simulink model "test_10gbe_mux_with_buffers"  (Simulink 6.2)
settings: Solver=ode45  StartTime=0.0  StopTime=4000  RelTol=1e-3
undefined symbols (not defined in the file): BEE2_usr
libraries: xbsIndex_r3 x551, xps_library x35, casper_library x16
(part 1 of 3)
settings Model: LastModifiedBy=dsp
settings DebuggingCC: SolverPrmCheckMsg=warning

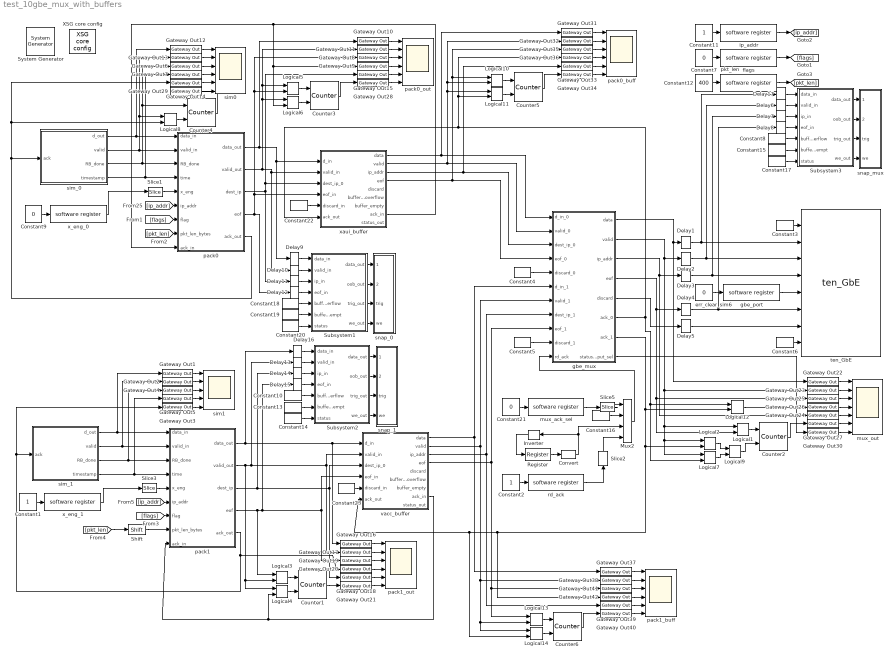
== system test_10gbe_mux_with_buffers ==
  " System Generator" : xbsIndex_r3/ System Generator  Tag=genX  xilinxfamily=Virtex2P  part=xc2vp70  speed=-7  package=ff1704  synthesis_tool=XST  directory=./test_mp_ub1/sysgen  testbench=off  simulink_period=1  sysclk_period=4.878  incr_netlist=off  trim_vbits=Everywhere in SubSystem  dbl_ovrd=According to Block Masks  core_generation=According to Block Masks  run_coregen=off  deprecated_control=off  eval_field=0
      settings: AttributesFormatString=System\nGenerator
  Constant1 : Constant
  Constant{3..5,8,10,13,15,18..19,22..23} (11 alike) : xbsIndex_r3/Constant  const=0  equ=P=C  arith_type=Boolean  n_bits=32  bin_pt=0  opselect=C  inp2=PCIN>>17  opr=+  inp1=P  carry=CIN  iostate=0  explicit_period=on  period=1  dbl_ovrd=off
  Constant11 : Constant
  Constant12 : Constant  Value=400
  Constant14 : xbsIndex_r3/Constant  const=0  equ=P=C  arith_type=Unsigned  n_bits=9  bin_pt=0  opselect=C  inp2=PCIN>>17  opr=+  inp1=P  carry=CIN  iostate=0  explicit_period=on  period=1  dbl_ovrd=off
  Constant16 : xbsIndex_r3/Constant  const=1  equ=P=C  arith_type=Boolean  n_bits=1  bin_pt=0  opselect=C  inp2=PCIN>>17  opr=+  inp1=P  carry=CIN  iostate=0  explicit_period=on  period=1  dbl_ovrd=off
  Constant17 : xbsIndex_r3/Constant  const=0  equ=P=C  arith_type=Unsigned  n_bits=9  bin_pt=0  opselect=C  inp2=PCIN>>17  opr=+  inp1=P  carry=CIN  iostate=0  explicit_period=on  period=1  dbl_ovrd=off
  Constant2 : Constant
  Constant20 : xbsIndex_r3/Constant  const=0  equ=P=C  arith_type=Unsigned  n_bits=9  bin_pt=0  opselect=C  inp2=PCIN>>17  opr=+  inp1=P  carry=CIN  iostate=0  explicit_period=on  period=1  dbl_ovrd=off
  Constant21 : Constant  Value=0
  Constant6 : xbsIndex_r3/Constant  const=1  equ=P=C  arith_type=Boolean  n_bits=32  bin_pt=0  opselect=C  inp2=PCIN>>17  opr=+  inp1=P  carry=CIN  iostate=0  explicit_period=on  period=1  dbl_ovrd=off
  Constant7 : Constant  Value=0
  Constant9 : Constant  Value=0
  Convert : xbsIndex_r3/Convert  arith_type=Boolean  n_bits=1  bin_pt=6  quantization=Truncate  overflow=Wrap  latency=0  explicit_period=off  period=1  dbl_ovrd=off  show_param=off  inserted_by_tool=off  pipeline=off
      settings: xl_area=[0, 0, 0, 0, 0, 0, 0]
  Counter{1..6} (6 alike) : xbsIndex_r3/Counter  cnt_type=Free Running  n_bits=8  bin_pt=0  arith_type=Unsigned  start_count=0  cnt_to=Inf  cnt_by_val=1  operation=Up  explicit_period=off  period=1  load_pin=off  rst=on  en=on  dbl_ovrd=off  show_param=off  use_rpm=on  gen_core=off
      settings: xl_area=[0, 0, 0, 0, 0, 0, 0]
  Delay{1..17} (17 alike) : xbsIndex_r3/Delay  latency=5  reg_retiming=on  explicit_period=off  period=1  en=off  accept_only_valid=off  init_zero=on  dbl_ovrd=off  show_param=off
      settings: xl_area=[0, 0, 0, 0, 0, 0, 0]
  Gateway Out{1..42} (42 alike) : xbsIndex_r3/Gateway Out  output_type=Double  nbits=8  bin_pt=6  arith_type=Boolean  quantization=Truncate  overflow=Wrap  hdl_port=on  timing_constraint=None  locs_specified=off  LOCs={}  needs_fixed_name=off  show_param=off
      settings: xl_area=[0, 0, 0, 0, 0, 0, 0]
  Inverter : xbsIndex_r3/Inverter  Orientation=left  latency=0  explicit_period=on  period=1  en=off  dbl_ovrd=off  show_param=off
      settings: xl_area=[0, 0, 0, 0, 0, 0, 0]
  Logical{1..8,10..11,13..14} (12 alike) : xbsIndex_r3/Logical  logical_function=AND  inputs=2  precision=Full  arith_type=Unsigned  n_bits=8  bin_pt=2  align_bp=on  latency=0  explicit_period=off  period=1  en=off  dbl_ovrd=off  show_param=off
      settings: xl_area=[0, 0, 0, 0, 0, 0, 0]
  Logical12 : xbsIndex_r3/Logical  logical_function=OR  inputs=2  precision=Full  arith_type=Unsigned  n_bits=8  bin_pt=2  align_bp=on  latency=0  explicit_period=off  period=1  en=off  dbl_ovrd=off  show_param=off
      settings: xl_area=[0, 0, 0, 0, 0, 0, 0]
  Logical9 : xbsIndex_r3/Logical  logical_function=OR  inputs=2  precision=Full  arith_type=Unsigned  n_bits=8  bin_pt=2  align_bp=on  latency=0  explicit_period=off  period=1  en=off  dbl_ovrd=off  show_param=off
      settings: xl_area=[0, 0, 0, 0, 0, 0, 0]
  Mux2 : xbsIndex_r3/Mux  inputs=3  precision=Full  arith_type="Signed  (2's comp)"  n_bits=8  bin_pt=2  quantization=Truncate  overflow=Wrap  latency=0  explicit_period=off  period=1  en=off  dbl_ovrd=off  show_param=off  mux_type=off  use_rpm=off  gen_core=off
      settings: xl_area=[0, 0, 0, 0, 0, 0, 0]
  Register : xbsIndex_r3/Register  init=0  reg_only_valid=off  explicit_period=on  period=1  rst=off  en=off  out_en=off  dbl_ovrd=off  show_param=off
      settings: xl_area=[0, 0, 0, 0, 0, 0, 0]
  Shift : xbsIndex_r3/Shift  shift_dir=Left  shift_bits=1  precision=User Defined  arith_type=Unsigned  n_bits=32  bin_pt=0  quantization=Truncate  overflow=Wrap  latency=0  explicit_period=off  period=1  en=off  dbl_ovrd=off  show_param=off
      settings: xl_area=[0, 0, 0, 0, 0, 0, 0]
  Slice1 : xbsIndex_r3/Slice  mode=Lower Bit Location + Width  nbits=16  bit1=0  base1=MSB of Input  bit0=0  base0=LSB of Input  boolean_output=off  explicit_period=off  period=1  dbl_ovrd=off
  Slice2 : xbsIndex_r3/Slice  Orientation=up  mode=Lower Bit Location + Width  nbits=1  bit1=0  base1=MSB of Input  bit0=0  base0=LSB of Input  boolean_output=on  explicit_period=off  period=1  dbl_ovrd=off
  Slice3 : xbsIndex_r3/Slice  mode=Lower Bit Location + Width  nbits=16  bit1=0  base1=MSB of Input  bit0=0  base0=LSB of Input  boolean_output=off  explicit_period=off  period=1  dbl_ovrd=off
  Slice5 : xbsIndex_r3/Slice  mode=Lower Bit Location + Width  nbits=2  bit1=0  base1=MSB of Input  bit0=0  base0=LSB of Input  boolean_output=off  explicit_period=off  period=1  dbl_ovrd=off
  Subsystem1 : Subsystem
  Subsystem2 : Subsystem
  Subsystem3 : Subsystem
  XSG core config : xps_library/XSG core config  Tag=xps:xsg  hw_sys=BEE2_usr  ibob_linux=off  clk_src=sys_clk2x  gpio_clk_io_group=iBOB:sma  gpio_clk_bit_index=0  clk_rate=205  sample_period=1  synthesis_tool=XST  mpc_type=powerpc405
  err_clear_sim6 : Constant  Value=0
  flags : xps_library/software register  Tag=xps:sw_reg  io_dir=From Processor  arith_type=Unsigned  bitwidth=32  bin_pt=0  sample_period=1  gw_name=test_10gbe_mux_with_buffers_flags_user_data_out
  gbe_mux : Subsystem  mask(mux_packets){max_packet_size_0=40, min_packet_size_0=20, max_packet_size_1=1500, min_packet_size_1=20}
      mask prompts: max_packet_size_0 "Input 0: Maximum single packet size (words)"; min_packet_size_0 "Input 0: Minimum single packet size (words)"; max_packet_size_1 "Input 1: Maximum single packet size (words)"; min_packet_size_1 "Input 1: Minimum single packet size (words)"
      mask help: This block allows you to mux together two data streams to be sent to the 10GbE core
  gbe_port : xps_library/software register  Tag=xps:sw_reg  io_dir=From Processor  arith_type=Unsigned  bitwidth=32  bin_pt=0  sample_period=1  gw_name=test_10gbe_mux_with_buffers_gbe_port_user_data_out
  ip_addr : xps_library/software register  Tag=xps:sw_reg  io_dir=From Processor  arith_type=Unsigned  bitwidth=32  bin_pt=0  sample_period=1  gw_name=test_10gbe_mux_with_buffers_ip_addr_user_data_out
  mux_ack_sel : xps_library/software register  Tag=xps:sw_reg  io_dir=From Processor  arith_type=Unsigned  bitwidth=32  bin_pt=0  sample_period=1  gw_name=test_10gbe_mux_with_buffers_mux_ack_sel_user_data_out
  mux_out : Scope  NumInputPorts=7
      settings: YMin=410.4~-1~-1~-1~0~-5~-5  YMax=453.6~1~1~1~1~5~5  SaveName=ScopeData10
  pack0 : Subsystem  mask{vector_len=100}
      mask prompts: vector_len "vector length"
  pack0_buff : Scope  NumInputPorts=6
      settings: YMin=410.4~-1~-1~-1~0~-5  YMax=453.6~1~1~1~1~5  SaveName=ScopeData16
  pack0_out : Scope  NumInputPorts=6
      settings: YMin=410.4~-1~-1~-1~0~-5  YMax=453.6~1~1~1~1~5  SaveName=ScopeData7
  pack1 : Subsystem  mask{vector_len=100}
      mask prompts: vector_len "vector length"
  pack1_buff : Scope  NumInputPorts=6
      settings: YMin=410.4~-1~-1~-1~0~-5  YMax=453.6~1~1~1~1~5  SaveName=ScopeData17
  pack1_out : Scope  NumInputPorts=6
      settings: YMin=410.4~-1~-1~-1~0~-5  YMax=453.6~1~1~1~1~5  SaveName=ScopeData11
  pkt_len : xps_library/software register  Tag=xps:sw_reg  io_dir=From Processor  arith_type=Unsigned  bitwidth=32  bin_pt=0  sample_period=1  gw_name=test_10gbe_mux_with_buffers_pkt_len_user_data_out
  rd_ack : xps_library/software register  Tag=xps:sw_reg  io_dir=From Processor  arith_type=Unsigned  bitwidth=32  bin_pt=0  sample_period=1  gw_name=test_10gbe_mux_with_buffers_rd_ack_user_data_out
  sim0 : Scope  NumInputPorts=6
      settings: YMin=410.4~-1~-1~-1~0~-5  YMax=453.6~1~1~1~1~5  SaveName=ScopeData2
  sim1 : Scope  NumInputPorts=5
      settings: YMin=95~0.95~-1~2~-1  YMax=105~1.05~1~3~1  SaveName=ScopeData12
  sim_0 : Subsystem
  sim_1 : Subsystem
  snap_0 : Subsystem  AncestorBlock=casper_library/Scopes/snap64  mask(snap64){nsamples=11}
      mask prompts: nsamples "No. of samples(2^?)"
      mask help:
      | The <i>snap</i> block provides a packaged solution to capturing data from
      | the FPGA fabric and making it accessible from the CPU.  The block comes in
      | 2 flavors: <i>snap</i> (which captures to a 32 bit wide Shared BRAM), and
      | <i>snap64</i> (which captures to 2x32 bit wide Shared BRAMs to effect a
      | 64 bit capture).
      mask Help: eval('xlWeb([getenv(''MLIB_ROOT''), ''\casper_library\doc\snap_usage.html''])')
  snap_1 : Subsystem  AncestorBlock=casper_library/Scopes/snap64  mask(snap64){nsamples=11}
      mask prompts: nsamples "No. of samples(2^?)"
      mask help:
      | The <i>snap</i> block provides a packaged solution to capturing data from
      | the FPGA fabric and making it accessible from the CPU.  The block comes in
      | 2 flavors: <i>snap</i> (which captures to a 32 bit wide Shared BRAM), and
      | <i>snap64</i> (which captures to 2x32 bit wide Shared BRAMs to effect a
      | 64 bit capture).
      mask Help: eval('xlWeb([getenv(''MLIB_ROOT''), ''\casper_library\doc\snap_usage.html''])')
  snap_mux : Subsystem  AncestorBlock=casper_library/Scopes/snap64  mask(snap64){nsamples=11}
      mask prompts: nsamples "No. of samples(2^?)"
      mask help:
      | The <i>snap</i> block provides a packaged solution to capturing data from
      | the FPGA fabric and making it accessible from the CPU.  The block comes in
      | 2 flavors: <i>snap</i> (which captures to a 32 bit wide Shared BRAM), and
      | <i>snap64</i> (which captures to 2x32 bit wide Shared BRAMs to effect a
      | 64 bit capture).
      mask Help: eval('xlWeb([getenv(''MLIB_ROOT''), ''\casper_library\doc\snap_usage.html''])')
  ten_GbE : xps_library/ten_GbE  Tag=xps:tengbe  port=BEE2_usr:2  mac_lite=on  show_param=off  pre_emph=3  swing=800
  vacc_buffer : Subsystem  mask(mux_packets){depth_data_bits=10, depth_hdr_bits=4}
      mask prompts: depth_data_bits "Depth contents (2^?)"; depth_hdr_bits "Maximum number of packets to buffer? (2^?)"
      mask help: This block allows you to mux together two data streams to be sent to the 10GbE core
      mask init:
      | fmtstr = sprintf('Max %d data words.\nMax %d pkts.', 2^depth_data_bits,2^depth_hdr_bits);
      | set_param(gcb, 'AttributesFormatString', fmtstr);
      settings: AttributesFormatString=|
      | Max 1024 data words.
      | Max 16 pkts.
  x_eng_0 : xps_library/software register  Tag=xps:sw_reg  io_dir=From Processor  arith_type=Unsigned  bitwidth=32  bin_pt=0  sample_period=1  gw_name=test_10gbe_mux_with_buffers_x_eng_0_user_data_out
  x_eng_1 : xps_library/software register  Tag=xps:sw_reg  io_dir=From Processor  arith_type=Unsigned  bitwidth=32  bin_pt=0  sample_period=1  gw_name=test_10gbe_mux_with_buffers_x_eng_1_user_data_out
  xaui_buffer : Subsystem  mask(mux_packets){depth_data_bits=10, depth_hdr_bits=4}
      mask prompts: depth_data_bits "Depth contents (2^?)"; depth_hdr_bits "Maximum number of packets to buffer? (2^?)"
      mask help: This block allows you to mux together two data streams to be sent to the 10GbE core
      mask init:
      | fmtstr = sprintf('Max %d data words.\nMax %d pkts.', 2^depth_data_bits,2^depth_hdr_bits);
      | set_param(gcb, 'AttributesFormatString', fmtstr);
      settings: AttributesFormatString=|
      | Max 1024 data words.
      | Max 16 pkts.
  wires:
  Slice1/1 -> pack0/5(x_eng)
  Constant12/1 -> pkt_len/1
  x_eng_0/1 -> Slice1/1
  Constant9/1 -> x_eng_0/1
  Constant11/1 -> ip_addr/1
  Constant7/1 -> flags/1
  pack0/1(data_out) -> Gateway Out10/1, Delay9/1, xaui_buffer/1(d_in)
  pack0/2(valid_out) -> Gateway Out11/1, Logical5/1, Logical6/1, Delay10/1, xaui_buffer/2(valid_in)
  pack0/3(dest_ip) -> Delay11/1, Gateway Out15/1, xaui_buffer/3(dest_ip_0)
  pack0/4(eof) -> Delay12/1, Gateway Out8/1, Logical5/2, xaui_buffer/4(eof_in)
  Subsystem1/1(data_out) -> snap_0/1(data_in)
  Subsystem1/2(oob_out) -> snap_0/2(oob_in)
  Subsystem1/3(trig_out) -> snap_0/3(trig)
  Subsystem1/4(we_out) -> snap_0/4(we)
  Constant18/1 -> Subsystem1/5(buffer_overflow)
  Constant19/1 -> Subsystem1/6(buffer_empt)
  Constant20/1 -> Subsystem1/7(status)
  Delay9/1 -> Subsystem1/1(data_in)
  Delay10/1 -> Subsystem1/2(valid_in)
  Delay11/1 -> Subsystem1/3(ip_in)
  Delay12/1 -> Subsystem1/4(eof_in)
  Subsystem2/1(data_out) -> snap_1/1(data_in)
  Subsystem2/2(oob_out) -> snap_1/2(oob_in)
  Subsystem2/3(trig_out) -> snap_1/3(trig)
  Subsystem2/4(we_out) -> snap_1/4(we)
  Constant10/1 -> Subsystem2/5(buffer_overflow)
  Constant13/1 -> Subsystem2/6(buffer_empt)
  Constant14/1 -> Subsystem2/7(status)
  Delay16/1 -> Subsystem2/1(data_in)
  Delay13/1 -> Subsystem2/2(valid_in)
  Delay14/1 -> Subsystem2/3(ip_in)
  Delay15/1 -> Subsystem2/4(eof_in)
  pack0/5(ack_out) -> sim_0/1(ack), Gateway Out14/1, Logical8/2
  sim_0/1(d_out) -> Gateway Out12/1, pack0/1(data_in)
  sim_0/2(valid) -> pack0/2(valid_in), Gateway Out13/1, Logical8/1
  sim_0/3(RB_done) -> pack0/3(RB_done), Gateway Out6/1, Counter4/1
  sim_0/4(timestamp) -> pack0/4(time), Gateway Out7/1
  sim_1/1(d_out) -> Gateway Out1/1, pack1/1(data_in)
  sim_1/2(valid) -> Gateway Out2/1, pack1/2(valid_in)
  sim_1/3(RB_done) -> Gateway Out4/1, pack1/3(RB_done)
  sim_1/4(timestamp) -> Gateway Out5/1, pack1/4(time)
  [ip_addr] -> pack0/6(ip_addr)
  ip_addr/1 -> [ip_addr]
  [flags] -> pack0/7(flag)
  flags/1 -> [flags]
  pkt_len/1 -> [pkt_len]
  [pkt_len] -> pack0/8(pkt_len_bytes)
  Slice3/1 -> pack1/5(x_eng)
  x_eng_1/1 -> Slice3/1
  Constant1/1 -> x_eng_1/1
  [ip_addr] -> pack1/6(ip_addr)
  [flags] -> pack1/7(flag)
  pack1/1(data_out) -> Delay16/1, Gateway Out16/1, vacc_buffer/1(d_in)
  pack1/2(valid_out) -> Delay13/1, Gateway Out17/1, vacc_buffer/2(valid_in), Logical3/2, Logical4/1
  pack1/3(dest_ip) -> Delay14/1, Gateway Out18/1, vacc_buffer/3(dest_ip_0)
  pack1/4(eof) -> Delay15/1, Gateway Out19/1, vacc_buffer/4(eof_in), Logical3/1
  pack1/5(ack_out) -> Gateway Out3/1, sim_1/1(ack), Gateway Out20/1
  Gateway Out12/1 -> sim0/1
  Gateway Out13/1 -> sim0/2
  Gateway Out6/1 -> sim0/3
  Gateway Out7/1 -> sim0/4
  Gateway Out14/1 -> sim0/5
  Gateway Out1/1 -> sim1/1
  Gateway Out2/1 -> sim1/2
  Gateway Out4/1 -> sim1/3
  Gateway Out5/1 -> sim1/4
  Gateway Out3/1 -> sim1/5
  Gateway Out10/1 -> pack0_out/1
  Gateway Out11/1 -> pack0_out/2
  Gateway Out8/1 -> pack0_out/3
  Gateway Out9/1 -> pack0_out/4
  Gateway Out15/1 -> pack0_out/5
  Gateway Out16/1 -> pack1_out/1
  Gateway Out17/1 -> pack1_out/2
  Gateway Out19/1 -> pack1_out/3
  Gateway Out20/1 -> pack1_out/4
  Gateway Out18/1 -> pack1_out/5
  Constant4/1 -> gbe_mux/5(discard_0)
  Constant5/1 -> gbe_mux/10(discard_1)
  gbe_mux/7(ack_1) -> Logical2/2, Gateway Out42/1, vacc_buffer/6(ack_out), Logical14/2, Logical12/2
  gbe_mux/6(ack_0) -> xaui_buffer/6(ack_out), Gateway Out36/1, Logical11/2, Logical7/2, Logical12/1
  Constant21/1 -> mux_ack_sel/1
  Slice5/1 -> Mux2/1
  mux_ack_sel/1 -> Slice5/1
  Mux2/1 -> gbe_mux/11(rd_ack)
  Register/1 -> Convert/1
  Inverter/1 -> Register/1
  Constant2/1 -> rd_ack/1
  rd_ack/1 -> Slice2/1
  Slice2/1 -> Mux2/4
  Convert/1 -> Inverter/1, Mux2/3
  Constant3/1 -> ten_GbE/1
  gbe_mux/1(data) -> Delay1/1, Gateway Out22/1
  gbe_mux/2(valid) -> Delay2/1, Gateway Out23/1, Logical1/1, Logical2/1, Logical7/1
  gbe_mux/3(ip_addr) -> Delay3/1, Gateway Out24/1
  gbe_mux/4(eof) -> Delay4/1, Gateway Out25/1, Logical1/2
  gbe_mux/5(discard) -> Delay5/1
  err_clear_sim6/1 -> gbe_port/1
  gbe_port/1 -> ten_GbE/5
  Constant6/1 -> ten_GbE/8
  Delay1/1 -> ten_GbE/2, Delay17/1
  Delay2/1 -> ten_GbE/3, Delay6/1
  Delay3/1 -> ten_GbE/4, Delay7/1
  Delay4/1 -> ten_GbE/6, Delay8/1
  Delay5/1 -> ten_GbE/7
  Subsystem3/1(data_out) -> snap_mux/1(data_in)
  Subsystem3/2(oob_out) -> snap_mux/2(oob_in)
  Subsystem3/3(trig_out) -> snap_mux/3(trig)
  Subsystem3/4(we_out) -> snap_mux/4(we)
  Constant8/1 -> Subsystem3/5(buffer_overflow)
  Constant15/1 -> Subsystem3/6(buffer_empt)
  Constant17/1 -> Subsystem3/7(status)
  Delay17/1 -> Subsystem3/1(data_in)
  Delay6/1 -> Subsystem3/2(valid_in)
  Delay7/1 -> Subsystem3/3(ip_in)
  Delay8/1 -> Subsystem3/4(eof_in)
  Constant16/1 -> Mux2/2
  Logical3/1 -> Counter1/1
  Logical4/1 -> Counter1/2
  Counter1/1 -> Gateway Out21/1
  Gateway Out21/1 -> pack1_out/6
  Gateway Out22/1 -> mux_out/1
  Gateway Out23/1 -> mux_out/2
  Gateway Out25/1 -> mux_out/3
  Gateway Out26/1 -> mux_out/4
  Gateway Out24/1 -> mux_out/5
  Logical1/1 -> Counter2/1
  Counter2/1 -> Gateway Out27/1
  Gateway Out27/1 -> mux_out/6
  Logical5/1 -> Counter3/1
  Logical6/1 -> Counter3/2
  Counter3/1 -> Gateway Out28/1
  Gateway Out28/1 -> pack0_out/6
  Logical8/1 -> Counter4/2
  Counter4/1 -> Gateway Out29/1
  Gateway Out29/1 -> sim0/6
  Gateway Out30/1 -> mux_out/7
  gbe_mux/8(status_input_sel) -> Gateway Out30/1
  Shift/1 -> pack1/8(pkt_len_bytes)
  [pkt_len] -> Shift/1
  Logical9/1 -> Counter2/2
  Logical2/1 -> Logical9/1
  Logical7/1 -> Logical9/2
  xaui_buffer/1(data) -> gbe_mux/1(d_in_0), Gateway Out31/1
  xaui_buffer/2(valid) -> gbe_mux/2(valid_0), Gateway Out32/1, Logical10/2, Logical11/1
  xaui_buffer/3(ip_addr) -> gbe_mux/3(dest_ip_0), Gateway Out33/1
  xaui_buffer/4(eof) -> gbe_mux/4(eof_0), Gateway Out35/1, Logical10/1
  Constant22/1 -> xaui_buffer/5(discard_in)
  xaui_buffer/8(ack_in) -> pack0/9(ack_in), Gateway Out9/1, Logical6/2
  vacc_buffer/1(data) -> gbe_mux/6(d_in_1), Gateway Out37/1
  vacc_buffer/2(valid) -> gbe_mux/7(valid_1), Gateway Out38/1, Logical13/2, Logical14/1
  vacc_buffer/3(ip_addr) -> gbe_mux/8(dest_ip_1), Gateway Out39/1
  vacc_buffer/4(eof) -> gbe_mux/9(eof_1), Gateway Out41/1, Logical13/1
  Constant23/1 -> vacc_buffer/5(discard_in)
  vacc_buffer/8(ack_in) -> Logical4/2, pack1/9(ack_in)
  Gateway Out31/1 -> pack0_buff/1
  Gateway Out32/1 -> pack0_buff/2
  Gateway Out35/1 -> pack0_buff/3
  Gateway Out36/1 -> pack0_buff/4
  Gateway Out33/1 -> pack0_buff/5
  Logical10/1 -> Counter5/1
  Logical11/1 -> Counter5/2
  Counter5/1 -> Gateway Out34/1
  Gateway Out34/1 -> pack0_buff/6
  Logical12/1 -> Gateway Out26/1
  Gateway Out37/1 -> pack1_buff/1
  Gateway Out38/1 -> pack1_buff/2
  Gateway Out41/1 -> pack1_buff/3
  Gateway Out42/1 -> pack1_buff/4
  Gateway Out39/1 -> pack1_buff/5
  Logical13/1 -> Counter6/1
  Logical14/1 -> Counter6/2
  Counter6/1 -> Gateway Out40/1
  Gateway Out40/1 -> pack1_buff/6

== system test_10gbe_mux_with_buffers/Subsystem1 ==
  data_in : Inport  Port=1  LatchInput=off
  valid_in : Inport  Port=2  LatchInput=off
  ip_in : Inport  Port=3  LatchInput=off
  eof_in : Inport  Port=4  LatchInput=off
  buffer_overflow : Inport  Port=5  LatchInput=off
  buffer_empt : Inport  Port=6  LatchInput=off
  status : Inport  Port=7  LatchInput=off
  Concat1 : xbsIndex_r3/Concat  num_inputs=5  explicit_period=off  period=1  dbl_ovrd=off
  Delay{1,4..6} (4 alike) : xbsIndex_r3/Delay  latency=2  reg_retiming=on  explicit_period=off  period=1  en=off  accept_only_valid=off  init_zero=on  dbl_ovrd=off  show_param=off
      settings: xl_area=[0, 0, 0, 0, 0, 0, 0]
  Logical4 : xbsIndex_r3/Logical  logical_function=AND  inputs=2  precision=Full  arith_type=Unsigned  n_bits=8  bin_pt=2  align_bp=on  latency=0  explicit_period=on  period=1  en=off  dbl_ovrd=off  show_param=off
      settings: xl_area=[0, 0, 0, 0, 0, 0, 0]
  Slice11 : xbsIndex_r3/Slice  mode=Lower Bit Location + Width  nbits=32-9-1-1-1  bit1=0  base1=MSB of Input  bit0=0  base0=LSB of Input  boolean_output=on  explicit_period=off  period=1  dbl_ovrd=off
  data_out : Outport
  oob_out : Outport  Port=2
  trig_out : Outport  Port=3
  we_out : Outport  Port=4
  wires:
  Slice11/1 -> Concat1/1
  Concat1/1 -> Delay4/1
  data_in/1 -> Delay1/1
  ip_in/1 -> Slice11/1
  Delay1/1 -> data_out/1
  Delay4/1 -> oob_out/1
  Delay5/1 -> Logical4/2, we_out/1
  Logical4/1 -> trig_out/1
  Delay6/1 -> Logical4/1
  valid_in/1 -> Delay5/1
  eof_in/1 -> Concat1/2, Delay6/1
  buffer_overflow/1 -> Concat1/3
  buffer_empt/1 -> Concat1/4
  status/1 -> Concat1/5

== system test_10gbe_mux_with_buffers/Subsystem2 ==
  data_in : Inport  Port=1  LatchInput=off
  valid_in : Inport  Port=2  LatchInput=off
  ip_in : Inport  Port=3  LatchInput=off
  eof_in : Inport  Port=4  LatchInput=off
  buffer_overflow : Inport  Port=5  LatchInput=off
  buffer_empt : Inport  Port=6  LatchInput=off
  status : Inport  Port=7  LatchInput=off
  Concat1 : xbsIndex_r3/Concat  num_inputs=5  explicit_period=off  period=1  dbl_ovrd=off
  Delay{1,4..6} (4 alike) : xbsIndex_r3/Delay  latency=2  reg_retiming=on  explicit_period=off  period=1  en=off  accept_only_valid=off  init_zero=on  dbl_ovrd=off  show_param=off
      settings: xl_area=[0, 0, 0, 0, 0, 0, 0]
  Logical4 : xbsIndex_r3/Logical  logical_function=AND  inputs=2  precision=Full  arith_type=Unsigned  n_bits=8  bin_pt=2  align_bp=on  latency=0  explicit_period=on  period=1  en=off  dbl_ovrd=off  show_param=off
      settings: xl_area=[0, 0, 0, 0, 0, 0, 0]
  Slice11 : xbsIndex_r3/Slice  mode=Lower Bit Location + Width  nbits=32-9-1-1-1  bit1=0  base1=MSB of Input  bit0=0  base0=LSB of Input  boolean_output=on  explicit_period=off  period=1  dbl_ovrd=off
  data_out : Outport
  oob_out : Outport  Port=2
  trig_out : Outport  Port=3
  we_out : Outport  Port=4
  wires:
  Slice11/1 -> Concat1/1
  Concat1/1 -> Delay4/1
  data_in/1 -> Delay1/1
  ip_in/1 -> Slice11/1
  Delay1/1 -> data_out/1
  Delay4/1 -> oob_out/1
  Delay5/1 -> Logical4/2, we_out/1
  Logical4/1 -> trig_out/1
  Delay6/1 -> Logical4/1
  valid_in/1 -> Delay5/1
  eof_in/1 -> Concat1/2, Delay6/1
  buffer_overflow/1 -> Concat1/3
  buffer_empt/1 -> Concat1/4
  status/1 -> Concat1/5

== system test_10gbe_mux_with_buffers/Subsystem3 ==
  data_in : Inport  Port=1  LatchInput=off
  valid_in : Inport  Port=2  LatchInput=off
  ip_in : Inport  Port=3  LatchInput=off
  eof_in : Inport  Port=4  LatchInput=off
  buffer_overflow : Inport  Port=5  LatchInput=off
  buffer_empt : Inport  Port=6  LatchInput=off
  status : Inport  Port=7  LatchInput=off
  Concat1 : xbsIndex_r3/Concat  num_inputs=5  explicit_period=off  period=1  dbl_ovrd=off
  Delay{1,4..6} (4 alike) : xbsIndex_r3/Delay  latency=2  reg_retiming=on  explicit_period=off  period=1  en=off  accept_only_valid=off  init_zero=on  dbl_ovrd=off  show_param=off
      settings: xl_area=[0, 0, 0, 0, 0, 0, 0]
  Logical4 : xbsIndex_r3/Logical  logical_function=AND  inputs=2  precision=Full  arith_type=Unsigned  n_bits=8  bin_pt=2  align_bp=on  latency=0  explicit_period=on  period=1  en=off  dbl_ovrd=off  show_param=off
      settings: xl_area=[0, 0, 0, 0, 0, 0, 0]
  Slice11 : xbsIndex_r3/Slice  mode=Lower Bit Location + Width  nbits=32-9-1-1-1  bit1=0  base1=MSB of Input  bit0=0  base0=LSB of Input  boolean_output=on  explicit_period=off  period=1  dbl_ovrd=off
  data_out : Outport
  oob_out : Outport  Port=2
  trig_out : Outport  Port=3
  we_out : Outport  Port=4
  wires:
  Slice11/1 -> Concat1/1
  Concat1/1 -> Delay4/1
  data_in/1 -> Delay1/1
  ip_in/1 -> Slice11/1
  Delay1/1 -> data_out/1
  Delay4/1 -> oob_out/1
  Delay5/1 -> Logical4/2, we_out/1
  Logical4/1 -> trig_out/1
  Delay6/1 -> Logical4/1
  valid_in/1 -> Delay5/1
  eof_in/1 -> Concat1/2, Delay6/1
  buffer_overflow/1 -> Concat1/3
  buffer_empt/1 -> Concat1/4
  status/1 -> Concat1/5

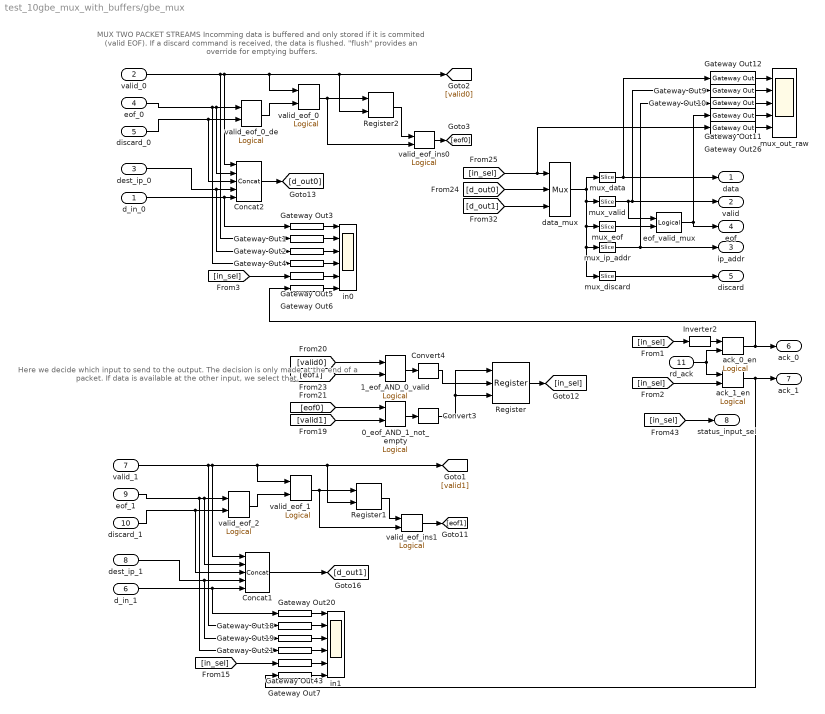
== system test_10gbe_mux_with_buffers/gbe_mux ==
  note: Here we decide which input
      | to send to the output.
      | The decision is only made at the end of a packet.
      | If data is available at the other input,
      | we select that.
  note: MUX TWO PACKET STREAMS
      | Incomming data is buffered and only stored if it is commited (valid EOF).
      | If a discard command is received, the data is flushed.
      | "flush" provides an override for emptying buffers.
  d_in_0 : Inport  Port=1  LatchInput=off
  valid_0 : Inport  Port=2  LatchInput=off
  dest_ip_0 : Inport  Port=3  LatchInput=off
  eof_0 : Inport  Port=4  LatchInput=off
  discard_0 : Inport  Port=5  LatchInput=off
  d_in_1 : Inport  Port=6  LatchInput=off
  valid_1 : Inport  Port=7  LatchInput=off
  dest_ip_1 : Inport  Port=8  LatchInput=off
  eof_1 : Inport  Port=9  LatchInput=off
  discard_1 : Inport  Port=10  LatchInput=off
  rd_ack : Inport  Port=11  LatchInput=off
  0_eof_AND_1_not_empty : xbsIndex_r3/Logical  logical_function=AND  inputs=2  precision=Full  arith_type=Unsigned  n_bits=8  bin_pt=2  align_bp=on  latency=0  explicit_period=on  period=1  en=off  dbl_ovrd=off  show_param=off
      settings: xl_area=[0, 0, 0, 0, 0, 0, 0]
  1_eof_AND_0_valid : xbsIndex_r3/Logical  logical_function=AND  inputs=2  precision=Full  arith_type=Unsigned  n_bits=8  bin_pt=2  align_bp=on  latency=0  explicit_period=on  period=1  en=off  dbl_ovrd=off  show_param=off
      settings: xl_area=[0, 0, 0, 0, 0, 0, 0]
  Concat1 : xbsIndex_r3/Concat  num_inputs=5  explicit_period=off  period=1  dbl_ovrd=off
  Concat2 : xbsIndex_r3/Concat  num_inputs=5  explicit_period=off  period=1  dbl_ovrd=off
  Convert3 : xbsIndex_r3/Convert  arith_type=Boolean  n_bits=8  bin_pt=6  quantization=Truncate  overflow=Wrap  latency=0  explicit_period=off  period=1  dbl_ovrd=off  show_param=off  inserted_by_tool=off  pipeline=off
      settings: xl_area=[0, 0, 0, 0, 0, 0, 0]
  Convert4 : xbsIndex_r3/Convert  arith_type=Boolean  n_bits=8  bin_pt=6  quantization=Truncate  overflow=Wrap  latency=0  explicit_period=off  period=1  dbl_ovrd=off  show_param=off  inserted_by_tool=off  pipeline=off
      settings: xl_area=[0, 0, 0, 0, 0, 0, 0]
  Gateway Out{1..7,9..12,18..21,26,43} (17 alike) : xbsIndex_r3/Gateway Out  output_type=Double  nbits=8  bin_pt=6  arith_type=Boolean  quantization=Truncate  overflow=Wrap  hdl_port=on  timing_constraint=None  locs_specified=off  LOCs={}  needs_fixed_name=off  show_param=off
      settings: xl_area=[0, 0, 0, 0, 0, 0, 0]
  Inverter2 : xbsIndex_r3/Inverter  latency=0  explicit_period=off  period=1  en=off  dbl_ovrd=off  show_param=off
      settings: xl_area=[0, 0, 0, 0, 0, 0, 0]
  Register : xbsIndex_r3/Register  init=0  reg_only_valid=off  explicit_period=on  period=1  rst=on  en=on  out_en=off  dbl_ovrd=off  show_param=off
      settings: xl_area=[0, 0, 0, 0, 0, 0, 0]
  Register1 : xbsIndex_r3/Register  init=1  reg_only_valid=off  explicit_period=off  period=1  rst=off  en=on  out_en=off  dbl_ovrd=off  show_param=off
      settings: xl_area=[0, 0, 0, 0, 0, 0, 0]
  Register2 : xbsIndex_r3/Register  init=0  reg_only_valid=off  explicit_period=off  period=1  rst=off  en=on  out_en=off  dbl_ovrd=off  show_param=off
      settings: xl_area=[0, 0, 0, 0, 0, 0, 0]
  ack_0_en : xbsIndex_r3/Logical  logical_function=AND  inputs=2  precision=Full  arith_type=Unsigned  n_bits=8  bin_pt=2  align_bp=on  latency=0  explicit_period=off  period=1  en=off  dbl_ovrd=off  show_param=off
      settings: xl_area=[0, 0, 0, 0, 0, 0, 0]
  ack_1_en : xbsIndex_r3/Logical  logical_function=AND  inputs=2  precision=Full  arith_type=Unsigned  n_bits=8  bin_pt=2  align_bp=on  latency=0  explicit_period=off  period=1  en=off  dbl_ovrd=off  show_param=off
      settings: xl_area=[0, 0, 0, 0, 0, 0, 0]
  data_mux : xbsIndex_r3/Mux  inputs=2  precision=Full  arith_type="Signed  (2's comp)"  n_bits=8  bin_pt=2  quantization=Truncate  overflow=Wrap  latency=0  explicit_period=off  period=1  en=off  dbl_ovrd=off  show_param=off  mux_type=off  use_rpm=off  gen_core=off
      settings: xl_area=[0, 0, 0, 0, 0, 0, 0]
  eof_valid_mux : xbsIndex_r3/Logical  logical_function=AND  inputs=2  precision=Full  arith_type=Unsigned  n_bits=8  bin_pt=2  align_bp=on  latency=0  explicit_period=off  period=1  en=off  dbl_ovrd=off  show_param=off
      settings: xl_area=[0, 0, 0, 0, 0, 0, 0]
  in0 : Scope  NumInputPorts=6
      settings: YMin=0~0~0~0~-5~-5  YMax=10000~1~10000~1~5~5  SaveName=ScopeData4
  in1 : Scope  NumInputPorts=6
      settings: YMin=0~0~0~0~-5~-5  YMax=10000~1~10000~1~5~5
  mux_data : xbsIndex_r3/Slice  mode=Lower Bit Location + Width  nbits=64  bit1=33  base1=LSB of Input  bit0=0  base0=LSB of Input  boolean_output=off  explicit_period=off  period=1  dbl_ovrd=off
  mux_discard : xbsIndex_r3/Slice  mode=Lower Bit Location + Width  nbits=1  bit1=0  base1=MSB of Input  bit0=96  base0=LSB of Input  boolean_output=on  explicit_period=off  period=1  dbl_ovrd=off
  mux_eof : xbsIndex_r3/Slice  mode=Upper Bit Location + Width  nbits=1  bit1=97  base1=LSB of Input  bit0=0  base0=LSB of Input  boolean_output=on  explicit_period=off  period=1  dbl_ovrd=off
  mux_ip_addr : xbsIndex_r3/Slice  mode=Lower Bit Location + Width  nbits=32  bit1=0  base1=MSB of Input  bit0=64  base0=LSB of Input  boolean_output=off  explicit_period=off  period=1  dbl_ovrd=off
  mux_out_raw : Scope  NumInputPorts=5
      settings: YMin=14.25~0.95~0.95~0.95~-1  YMax=15.75~1.05~1.05~1.05~1  SaveName=ScopeData5
  mux_valid : xbsIndex_r3/Slice  mode=Lower Bit Location + Width  nbits=1  bit1=0  base1=MSB of Input  bit0=98  base0=LSB of Input  boolean_output=on  explicit_period=off  period=1  dbl_ovrd=off
  valid_eof_0 : xbsIndex_r3/Logical  logical_function=AND  inputs=2  precision=Full  arith_type=Unsigned  n_bits=8  bin_pt=2  align_bp=on  latency=0  explicit_period=on  period=1  en=off  dbl_ovrd=off  show_param=off
      settings: xl_area=[0, 0, 0, 0, 0, 0, 0]
  valid_eof_0_de : xbsIndex_r3/Logical  logical_function=OR  inputs=2  precision=Full  arith_type=Unsigned  n_bits=8  bin_pt=2  align_bp=on  latency=0  explicit_period=on  period=1  en=off  dbl_ovrd=off  show_param=off
      settings: xl_area=[0, 0, 0, 0, 0, 0, 0]
  valid_eof_1 : xbsIndex_r3/Logical  logical_function=AND  inputs=2  precision=Full  arith_type=Unsigned  n_bits=8  bin_pt=2  align_bp=on  latency=0  explicit_period=on  period=1  en=off  dbl_ovrd=off  show_param=off
      settings: xl_area=[0, 0, 0, 0, 0, 0, 0]
  valid_eof_2 : xbsIndex_r3/Logical  logical_function=OR  inputs=2  precision=Full  arith_type=Unsigned  n_bits=8  bin_pt=2  align_bp=on  latency=0  explicit_period=on  period=1  en=off  dbl_ovrd=off  show_param=off
      settings: xl_area=[0, 0, 0, 0, 0, 0, 0]
  valid_eof_ins0 : xbsIndex_r3/Logical  logical_function=OR  inputs=2  precision=Full  arith_type=Unsigned  n_bits=8  bin_pt=2  align_bp=on  latency=0  explicit_period=off  period=1  en=off  dbl_ovrd=off  show_param=off
      settings: xl_area=[0, 0, 0, 0, 0, 0, 0]
  valid_eof_ins1 : xbsIndex_r3/Logical  logical_function=OR  inputs=2  precision=Full  arith_type=Unsigned  n_bits=8  bin_pt=2  align_bp=on  latency=0  explicit_period=off  period=1  en=off  dbl_ovrd=off  show_param=off
      settings: xl_area=[0, 0, 0, 0, 0, 0, 0]
  data : Outport
  valid : Outport  Port=2
  ip_addr : Outport  Port=3
  eof : Outport  Port=4
  discard : Outport  Port=5
  ack_0 : Outport  Port=6
  ack_1 : Outport  Port=7
  status_input_sel : Outport  Port=8
  wires:
  valid_1/1 -> Gateway Out18/1, valid_eof_1/1, Register1/2, [valid1], Concat1/1
  0_eof_AND_1_not_empty/1 -> Convert3/1
  1_eof_AND_0_valid/1 -> Convert4/1
  Convert3/1 -> Register/3, Register/1
  Convert4/1 -> Register/2
  Gateway Out12/1 -> mux_out_raw/1
  Gateway Out9/1 -> mux_out_raw/2
  Gateway Out10/1 -> mux_out_raw/3
  Gateway Out11/1 -> mux_out_raw/4
  [valid1] -> 0_eof_AND_1_not_empty/2
  [valid0] -> 1_eof_AND_0_valid/1
  [eof0] -> 0_eof_AND_1_not_empty/1
  [eof1] -> 1_eof_AND_0_valid/2
  [in_sel] -> data_mux/1, Gateway Out26/1
  [d_out0] -> data_mux/2
  [d_out1] -> data_mux/3
  [in_sel] -> status_input_sel/1
  valid_eof_1/1 -> Register1/1, valid_eof_ins1/2
  Concat1/1 -> [d_out1]
  data_mux/1 -> mux_ip_addr/1, mux_discard/1, mux_eof/1, mux_valid/1, mux_data/1
  mux_data/1 -> Gateway Out12/1, data/1
  mux_valid/1 -> eof_valid_mux/1, Gateway Out9/1, valid/1
  mux_ip_addr/1 -> Gateway Out10/1, ip_addr/1
  eof_valid_mux/1 -> Gateway Out11/1, eof/1
  mux_eof/1 -> eof_valid_mux/2
  Gateway Out20/1 -> in1/1
  Gateway Out18/1 -> in1/2
  Gateway Out19/1 -> in1/3
  Gateway Out21/1 -> in1/4
  Gateway Out26/1 -> mux_out_raw/5
  Register/1 -> [in_sel]
  [in_sel] -> Gateway Out43/1
  Gateway Out43/1 -> in1/5
  eof_1/1 -> valid_eof_2/1, Concat1/2, Gateway Out21/1
  discard_1/1 -> valid_eof_2/2, Concat1/3
  valid_eof_2/1 -> valid_eof_1/2
  ack_0_en/1 -> ack_0/1, Gateway Out6/1
  ack_1_en/1 -> ack_1/1, Gateway Out7/1
  rd_ack/1 -> ack_0_en/2, ack_1_en/1
  [in_sel] -> ack_1_en/2
  Inverter2/1 -> ack_0_en/1
  [in_sel] -> Inverter2/1
  dest_ip_1/1 -> Gateway Out19/1, Concat1/4
  d_in_1/1 -> Gateway Out20/1, Concat1/5
  valid_0/1 -> Gateway Out1/1, valid_eof_0/1, Register2/2, [valid0], Concat2/1
  valid_eof_0/1 -> Register2/1, valid_eof_ins0/2
  Concat2/1 -> [d_out0]
  Gateway Out3/1 -> in0/1
  Gateway Out1/1 -> in0/2
  Gateway Out2/1 -> in0/3
  Gateway Out4/1 -> in0/4
  [in_sel] -> Gateway Out5/1
  Gateway Out5/1 -> in0/5
  eof_0/1 -> valid_eof_0_de/1, Concat2/2, Gateway Out4/1
  discard_0/1 -> valid_eof_0_de/2, Concat2/3
  valid_eof_0_de/1 -> valid_eof_0/2
  dest_ip_0/1 -> Gateway Out2/1, Concat2/4
  d_in_0/1 -> Gateway Out3/1, Concat2/5
  mux_discard/1 -> discard/1
  Gateway Out6/1 -> in0/6
  Gateway Out7/1 -> in1/6
  valid_eof_ins1/1 -> [eof1]
  Register1/1 -> valid_eof_ins1/1
  Register2/1 -> valid_eof_ins0/1
  valid_eof_ins0/1 -> [eof0]

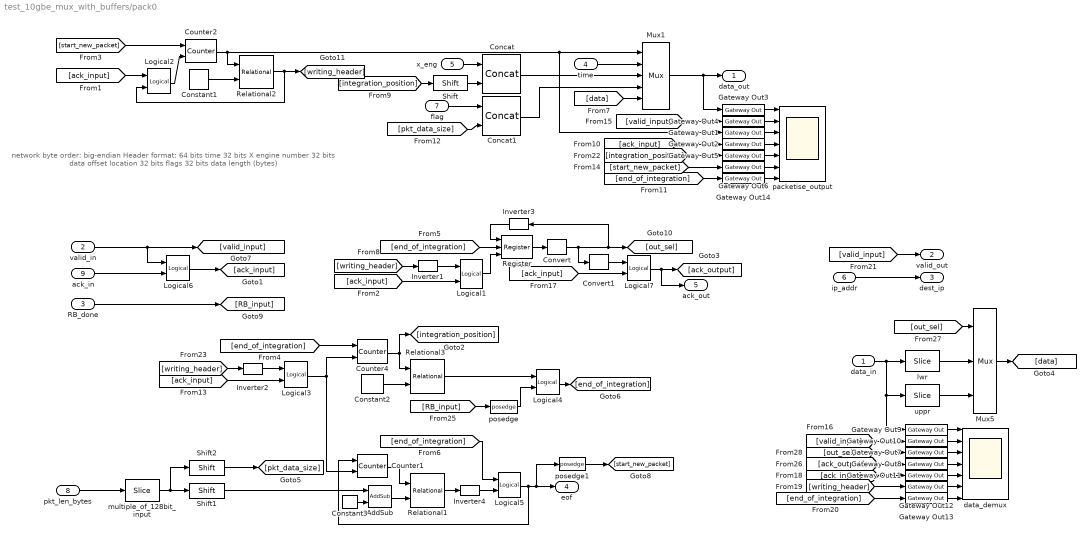
== system test_10gbe_mux_with_buffers/pack0 ==
  note: network byte order: big-endian
      |
      | Header format:
      | 64 bits time
      | 32 bits X engine number
      | 32 bits data offset location
      | 32 bits flags
      | 32 bits data length (bytes)
  data_in : Inport  Port=1  LatchInput=off
  valid_in : Inport  Port=2  LatchInput=off
  RB_done : Inport  Port=3  LatchInput=off
  time : Inport  Port=4  LatchInput=off
  x_eng : Inport  Port=5  LatchInput=off
  ip_addr : Inport  Port=6  LatchInput=off
  flag : Inport  Port=7  LatchInput=off
  pkt_len_bytes : Inport  Port=8  LatchInput=off
  ack_in : Inport  Port=9  LatchInput=off
  AddSub : xbsIndex_r3/AddSub  mode=Subtraction  precision=Full  arith_type=Unsigned  n_bits=8  bin_pt=2  quantization=Truncate  overflow=Wrap  latency=0  explicit_period=on  period=1  use_carryin=off  use_carryout=off  en=off  dbl_ovrd=off  show_param=off  use_core=on  pipeline=off  use_rpm=on  gen_core=off
      settings: xl_area=[0, 0, 0, 0, 0, 0, 0]
  Concat : xbsIndex_r3/Concat  num_inputs=2  explicit_period=off  period=1  dbl_ovrd=off
  Concat1 : xbsIndex_r3/Concat  num_inputs=2  explicit_period=off  period=1  dbl_ovrd=off
  Constant1 : xbsIndex_r3/Constant  const=2  equ=P=C  arith_type=Unsigned  n_bits=2  bin_pt=0  opselect=C  inp2=PCIN>>17  opr=+  inp1=P  carry=CIN  iostate=0  explicit_period=off  period=1  dbl_ovrd=off
  Constant2 : xbsIndex_r3/Constant  const=2*vector_len-1  equ=P=C  arith_type=Unsigned  n_bits=32  bin_pt=0  opselect=C  inp2=PCIN>>17  opr=+  inp1=P  carry=CIN  iostate=0  explicit_period=off  period=1  dbl_ovrd=off
  Constant3 : xbsIndex_r3/Constant  const=2  equ=P=C  arith_type=Unsigned  n_bits=32  bin_pt=0  opselect=C  inp2=PCIN>>17  opr=+  inp1=P  carry=CIN  iostate=0  explicit_period=off  period=1  dbl_ovrd=off
  Convert : xbsIndex_r3/Convert  arith_type=Unsigned  n_bits=1  bin_pt=0  quantization=Truncate  overflow=Wrap  latency=0  explicit_period=off  period=1  dbl_ovrd=off  show_param=off  inserted_by_tool=off  pipeline=off
      settings: xl_area=[0, 0, 0, 0, 0, 0, 0]
  Convert1 : xbsIndex_r3/Convert  arith_type=Boolean  n_bits=1  bin_pt=0  quantization=Truncate  overflow=Wrap  latency=0  explicit_period=off  period=1  dbl_ovrd=off  show_param=off  inserted_by_tool=off  pipeline=off
      settings: xl_area=[0, 0, 0, 0, 0, 0, 0]
  Counter1 : xbsIndex_r3/Counter  cnt_type=Free Running  n_bits=32  bin_pt=0  arith_type=Unsigned  start_count=0  cnt_to=1023  cnt_by_val=1  operation=Up  explicit_period=on  period=1  load_pin=off  rst=on  en=on  dbl_ovrd=off  show_param=off  use_rpm=on  gen_core=off
      settings: xl_area=[0, 0, 0, 0, 0, 0, 0]
  Counter2 : xbsIndex_r3/Counter  cnt_type=Free Running  n_bits=2  bin_pt=0  arith_type=Unsigned  start_count=0  cnt_to=1023  cnt_by_val=1  operation=Up  explicit_period=on  period=1  load_pin=off  rst=on  en=on  dbl_ovrd=off  show_param=off  use_rpm=on  gen_core=off
      settings: xl_area=[0, 0, 0, 0, 0, 0, 0]
  Counter4 : xbsIndex_r3/Counter  cnt_type=Free Running  n_bits=32  bin_pt=0  arith_type=Unsigned  start_count=0  cnt_to=1023  cnt_by_val=1  operation=Up  explicit_period=on  period=1  load_pin=off  rst=on  en=on  dbl_ovrd=off  show_param=off  use_rpm=on  gen_core=off
      settings: xl_area=[0, 0, 0, 0, 0, 0, 0]
  Gateway Out{1..14} (14 alike) : xbsIndex_r3/Gateway Out  output_type=Double  nbits=8  bin_pt=6  arith_type=Boolean  quantization=Truncate  overflow=Wrap  hdl_port=on  timing_constraint=None  locs_specified=off  LOCs={}  needs_fixed_name=off  show_param=off
      settings: xl_area=[0, 0, 0, 0, 0, 0, 0]
  Inverter1 : xbsIndex_r3/Inverter  latency=0  explicit_period=off  period=1  en=off  dbl_ovrd=off  show_param=off
      settings: xl_area=[0, 0, 0, 0, 0, 0, 0]
  Inverter2 : xbsIndex_r3/Inverter  latency=0  explicit_period=off  period=1  en=off  dbl_ovrd=off  show_param=off
      settings: xl_area=[0, 0, 0, 0, 0, 0, 0]
  Inverter3 : xbsIndex_r3/Inverter  Orientation=left  latency=0  explicit_period=on  period=1  en=off  dbl_ovrd=off  show_param=off
      settings: xl_area=[0, 0, 0, 0, 0, 0, 0]
  Inverter4 : xbsIndex_r3/Inverter  latency=0  explicit_period=off  period=1  en=off  dbl_ovrd=off  show_param=off
      settings: xl_area=[0, 0, 0, 0, 0, 0, 0]
  Logical{1..3,6..7} (5 alike) : xbsIndex_r3/Logical  logical_function=AND  inputs=2  precision=Full  arith_type=Unsigned  n_bits=8  bin_pt=2  align_bp=on  latency=0  explicit_period=off  period=1  en=off  dbl_ovrd=off  show_param=off
      settings: xl_area=[0, 0, 0, 0, 0, 0, 0]
  Logical4 : xbsIndex_r3/Logical  logical_function=OR  inputs=2  precision=Full  arith_type=Unsigned  n_bits=8  bin_pt=2  align_bp=on  latency=0  explicit_period=off  period=1  en=off  dbl_ovrd=off  show_param=off
      settings: xl_area=[0, 0, 0, 0, 0, 0, 0]
  Logical5 : xbsIndex_r3/Logical  logical_function=OR  inputs=2  precision=Full  arith_type=Unsigned  n_bits=8  bin_pt=2  align_bp=on  latency=0  explicit_period=off  period=1  en=off  dbl_ovrd=off  show_param=off
      settings: xl_area=[0, 0, 0, 0, 0, 0, 0]
  Mux1 : xbsIndex_r3/Mux  inputs=4  precision=Full  arith_type="Signed  (2's comp)"  n_bits=8  bin_pt=2  quantization=Truncate  overflow=Wrap  latency=0  explicit_period=off  period=1  en=off  dbl_ovrd=off  show_param=off  mux_type=off  use_rpm=off  gen_core=off
      settings: xl_area=[0, 0, 0, 0, 0, 0, 0]
  Mux5 : xbsIndex_r3/Mux  inputs=2  precision=Full  arith_type="Signed  (2's comp)"  n_bits=8  bin_pt=2  quantization=Truncate  overflow=Wrap  latency=0  explicit_period=on  period=1  en=off  dbl_ovrd=off  show_param=off  mux_type=off  use_rpm=off  gen_core=off
      settings: xl_area=[0, 0, 0, 0, 0, 0, 0]
  Register : xbsIndex_r3/Register  init=0  reg_only_valid=off  explicit_period=on  period=1  rst=on  en=on  out_en=off  dbl_ovrd=off  show_param=off
      settings: xl_area=[0, 0, 0, 0, 0, 0, 0]
  Relational1 : xbsIndex_r3/Relational  mode=a<=b  latency=0  explicit_period=off  period=1  en=off  dbl_ovrd=off  show_param=off
      settings: xl_area=[0, 0, 0, 0, 0, 0, 0]
  Relational2 : xbsIndex_r3/Relational  mode=a<=b  latency=0  explicit_period=off  period=1  en=off  dbl_ovrd=off  show_param=off
      settings: xl_area=[0, 0, 0, 0, 0, 0, 0]
  Relational3 : xbsIndex_r3/Relational  mode=a>=b  latency=0  explicit_period=off  period=1  en=off  dbl_ovrd=off  show_param=off
      settings: xl_area=[0, 0, 0, 0, 0, 0, 0]
  Shift : xbsIndex_r3/Shift  shift_dir=Left  shift_bits=3  precision=Full  arith_type="Signed  (2's comp)"  n_bits=8  bin_pt=2  quantization=Truncate  overflow=Wrap  latency=0  explicit_period=off  period=1  en=off  dbl_ovrd=off  show_param=off
      settings: xl_area=[0, 0, 0, 0, 0, 0, 0]
  Shift1 : xbsIndex_r3/Shift  shift_dir=Left  shift_bits=1  precision=Full  arith_type="Signed  (2's comp)"  n_bits=8  bin_pt=2  quantization=Truncate  overflow=Wrap  latency=0  explicit_period=off  period=1  en=off  dbl_ovrd=off  show_param=off
      settings: xl_area=[0, 0, 0, 0, 0, 0, 0]
  Shift2 : xbsIndex_r3/Shift  shift_dir=Left  shift_bits=4  precision=Full  arith_type="Signed  (2's comp)"  n_bits=8  bin_pt=2  quantization=Truncate  overflow=Wrap  latency=0  explicit_period=off  period=1  en=off  dbl_ovrd=off  show_param=off
      settings: xl_area=[0, 0, 0, 0, 0, 0, 0]
  data_demux : Scope  NumInputPorts=7
      settings: YMin=410.4~-1~-1~-1~0~-5~-5  YMax=453.6~1~1~1~1~5~5  SaveName=ScopeData3
  lwr : xbsIndex_r3/Slice  mode=Lower Bit Location + Width  nbits=64  bit1=0  base1=MSB of Input  bit0=0  base0=LSB of Input  boolean_output=off  explicit_period=off  period=1  dbl_ovrd=off
  multiple_of_128bit_input : xbsIndex_r3/Slice  mode=Two Bit Locations  nbits=64  bit1=0  base1=MSB of Input  bit0=4  base0=LSB of Input  boolean_output=off  explicit_period=off  period=1  dbl_ovrd=off
  packetise_output : Scope  NumInputPorts=7
      settings: YMin=410.4~-1~-1~-1~0~-5~-5  YMax=453.6~1~1~1~1~5~5
  posedge : casper_library/Misc/posedge  Tag=Rising Edge Detector
  posedge1 : casper_library/Misc/posedge  Tag=Rising Edge Detector
  uppr : xbsIndex_r3/Slice  mode=Upper Bit Location + Width  nbits=64  bit1=0  base1=MSB of Input  bit0=0  base0=LSB of Input  boolean_output=off  explicit_period=off  period=1  dbl_ovrd=off
  data_out : Outport
  valid_out : Outport  Port=2
  dest_ip : Outport  Port=3
  eof : Outport  Port=4
  ack_out : Outport  Port=5
  wires:
  lwr/1 -> Mux5/2
  uppr/1 -> Mux5/3
  [ack_input] -> Logical1/2
  Counter1/1 -> Relational1/1
  Logical5/1 -> Counter1/1, eof/1, posedge1/1
  Constant1/1 -> Relational2/2
  Counter2/1 -> Relational2/1, Mux1/1, Gateway Out1/1
  time/1 -> Mux1/2
  Logical2/1 -> Counter2/2
  Relational2/1 -> Logical2/2, [writing_header]
  [ack_input] -> Logical2/1
  [start_new_packet] -> Counter2/1
  [end_of_integration] -> Counter4/1
  Counter4/1 -> [integration_position], Relational3/1
  Mux1/1 -> data_out/1, Gateway Out3/1
  Mux5/1 -> [data]
  [writing_header] -> Inverter1/1
  Inverter1/1 -> Logical1/1
  x_eng/1 -> Concat/1
  [integration_position] -> Shift/1
  Concat/1 -> Mux1/3
  valid_in/1 -> [valid_input], Logical6/1
  ip_addr/1 -> dest_ip/1
  flag/1 -> Concat1/1
  [pkt_data_size] -> Concat1/2
  Concat1/1 -> Mux1/4
  Logical3/1 -> Counter4/2, Counter1/2
  Gateway Out3/1 -> packetise_output/1
  Gateway Out4/1 -> packetise_output/2
  Gateway Out1/1 -> packetise_output/3
  Gateway Out2/1 -> packetise_output/4
  Gateway Out5/1 -> packetise_output/5
  Gateway Out6/1 -> packetise_output/6
  [data] -> Mux1/5
  Relational1/1 -> Inverter4/1
  [end_of_integration] -> Logical5/1
  Logical6/1 -> [ack_input]
  ack_in/1 -> Logical6/2
  [start_new_packet] -> Gateway Out6/1
  [valid_input] -> Gateway Out4/1
  Gateway Out9/1 -> data_demux/1
  Gateway Out10/1 -> data_demux/2
  Gateway Out7/1 -> data_demux/3
  Gateway Out8/1 -> data_demux/4
  Gateway Out11/1 -> data_demux/5
  Gateway Out12/1 -> data_demux/6
  [valid_input] -> Gateway Out10/1
  Register/1 -> Convert/1
  Inverter3/1 -> Register/1
  [ack_input] -> Logical7/2
  Logical7/1 -> [ack_output], ack_out/1
  Convert1/1 -> Logical7/1
  [ack_input] -> Gateway Out11/1
  [writing_header] -> Gateway Out12/1
  Gateway Out13/1 -> data_demux/7
  [end_of_integration] -> Gateway Out13/1
  data_in/1 -> lwr/1, uppr/1, Gateway Out9/1
  [valid_input] -> valid_out/1
  Convert/1 -> Inverter3/1, [out_sel], Convert1/1
  Constant2/1 -> Relational3/2
  Gateway Out14/1 -> packetise_output/7
  [end_of_integration] -> Gateway Out14/1
  Shift/1 -> Concat/2
  Logical4/1 -> [end_of_integration]
  Relational3/1 -> Logical4/1
  posedge/1 -> Logical4/2
  [integration_position] -> Gateway Out5/1
  Logical1/1 -> Register/3
  [end_of_integration] -> Register/2
  [ack_input] -> Logical3/2
  [writing_header] -> Inverter2/1
  Inverter2/1 -> Logical3/1
  Inverter4/1 -> Logical5/2
  pkt_len_bytes/1 -> multiple_of_128bit_input/1
  multiple_of_128bit_input/1 -> Shift1/1, Shift2/1
  Shift1/1 -> AddSub/1
  AddSub/1 -> Relational1/2
  Constant3/1 -> AddSub/2
  Shift2/1 -> [pkt_data_size]
  posedge1/1 -> [start_new_packet]
  [ack_input] -> Gateway Out2/1
  RB_done/1 -> [RB_input]
  [RB_input] -> posedge/1
  [ack_output] -> Gateway Out8/1
  [out_sel] -> Mux5/1
  [out_sel] -> Gateway Out7/1
